simulink subsystem "Motores"  (R2023b)
settings: Solver=VariableStepAuto  StartTime=0.0  StopTime=10.0  RelTol=1e-3
libraries: arduinolib x6, simulink x2
settings Model: Creator=Andrés  LastModifiedBy=Andrés

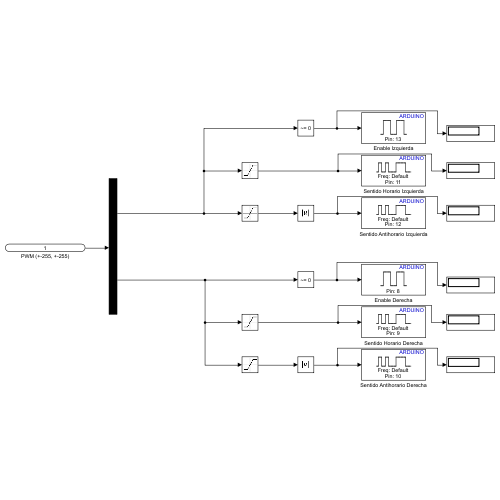
[thumbnail: Simulink's stored preview of the top-level diagram]
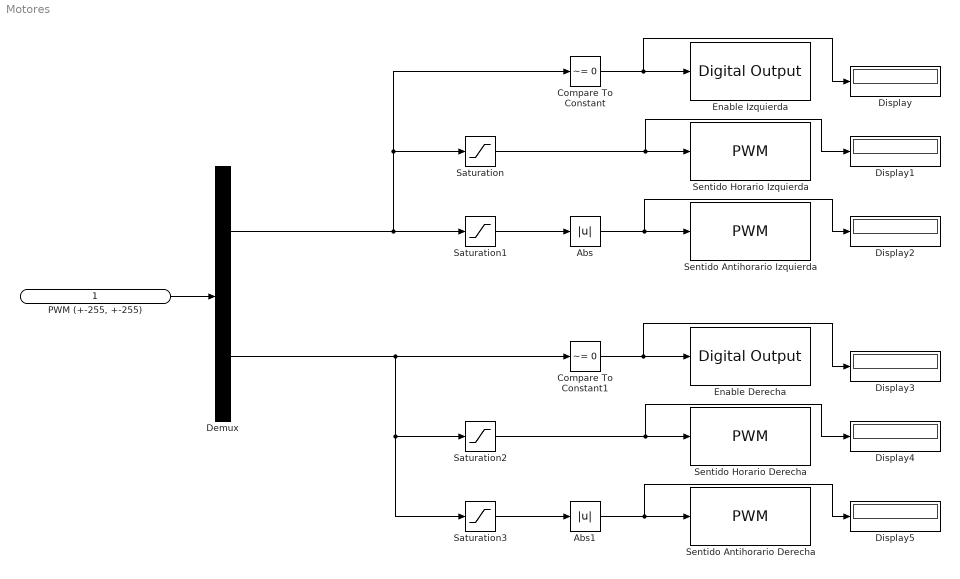
== system Motores ==
  "PWM (+-255, +-255)" : Inport
  Abs : Abs  SaturateOnIntegerOverflow=off
  Abs1 : Abs  SaturateOnIntegerOverflow=off
  Compare To Constant : simulink/Logic and Bit Operations/Compare To Constant  relop=~=  const=0  OutDataTypeStr=boolean
  Compare To Constant1 : simulink/Logic and Bit Operations/Compare To Constant  relop=~=  const=0  OutDataTypeStr=boolean
  Demux : Demux  Outputs=2
  Display{,1..5} (6 alike) : Display
  Enable Derecha : arduinolib/Digital Output  pinNumber=8  Direction=output  blockPlatform=arduino
  Enable Izquierda : arduinolib/Digital Output  pinNumber=13  Direction=output  blockPlatform=arduino
  Saturation : Saturate  UpperLimit=255  LowerLimit=0
  Saturation1 : Saturate  UpperLimit=0  LowerLimit=-255
  Saturation2 : Saturate  UpperLimit=255  LowerLimit=0
  Saturation3 : Saturate  UpperLimit=2  LowerLimit=-255
  Sentido Antihorario Derecha : arduinolib/PWM  pinNumber=10  frequencyType=Default  desiredFrequency=490.2  achievableFrequency=490.2
  Sentido Antihorario Izquierda : arduinolib/PWM  pinNumber=12  frequencyType=Default  desiredFrequency=490.2  achievableFrequency=490.2
  Sentido Horario Derecha : arduinolib/PWM  pinNumber=9  frequencyType=Default  desiredFrequency=490.2  achievableFrequency=490.2
  Sentido Horario Izquierda : arduinolib/PWM  pinNumber=11  frequencyType=Default  desiredFrequency=490.2  achievableFrequency=490.2
  wires:
  Demux/2 -> Compare To Constant1/1, Saturation2/1, Saturation3/1
  Abs1/1 -> Sentido Antihorario Derecha/1, Display5/1
  Compare To Constant1/1 -> Enable Derecha/1, Display3/1
  Compare To Constant/1 -> Enable Izquierda/1, Display/1
  Saturation3/1 -> Abs1/1
  Saturation/1 -> Display1/1, Sentido Horario Izquierda/1
  Saturation2/1 -> Display4/1, Sentido Horario Derecha/1
  Abs/1 -> Sentido Antihorario Izquierda/1, Display2/1
  Demux/1 -> Saturation1/1, Saturation/1, Compare To Constant/1
  Saturation1/1 -> Abs/1
  "PWM (+-255, +-255)"/1 -> Demux/1
